simulink model "AGS_TFM_modelo_Aire_PI_descentralizado_clasico"  (R2025b)
settings: Solver=ode23tb  StartTime=0.0  StopTime=320  MaxStep=0.05  RelTol=1e-3
values from neighbouring files (symbols this model uses):
  k_Faraday_air = N_cells * M_O2 / (4 * F * Y_O2_air)    (= 0.000128302952219)    [AGS_base_subsitema_aire_SIMULINK.m]
  k_mref = lambda_air * k_Faraday_air    (= 0.000230945313994)    [AGS_base_subsitema_aire_SIMULINK.m]
  k_stack = 1.56e6    (= 1560000)    [AGS_base_subsitema_aire_SIMULINK.m]
  k_valve_max = 4e-4    (= 0.0004)    [AGS_base_subsitema_aire_SIMULINK.m]
  mdot_table_gs = [mdot_0_gs;mdot_40_tab; mdot_60_tab;          mdot_80_tab; mdot_100_tab; mdot_120_tab]    [AGS_init_mapa_compresor_2D.m]
  N_bp = [0 40000 60000 80000 100000 120000]    [AGS_init_mapa_compresor_2D.m]
  p_amb = 101325    [AGS_base_subsitema_aire_SIMULINK.m]
  PR_bp = 1.00:0.025:3.50    [AGS_init_mapa_compresor_2D.m]
  R_air = 287    [AGS_base_subsitema_aire_SIMULINK.m]
  T_air = 298.15    [AGS_base_subsitema_aire_SIMULINK.m]
  tau_N = 2.0 / 2.303    (= 0.868432479375)    [AGS_base_subsitema_aire_SIMULINK.m]
  V_eq = 0.01664    [AGS_base_subsitema_aire_SIMULINK.m]
libraries: slpidlib x2
settings Model: SimulationMode=accelerator  Creator=agonz  LastModifiedBy=agonz
settings DataIOCC: SaveOutput=off

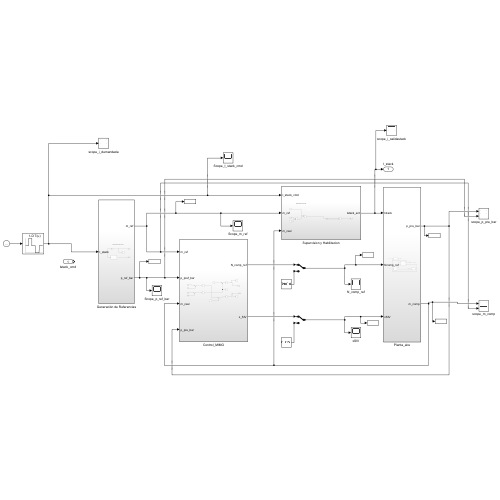
[thumbnail: Simulink's stored preview of the top-level diagram]
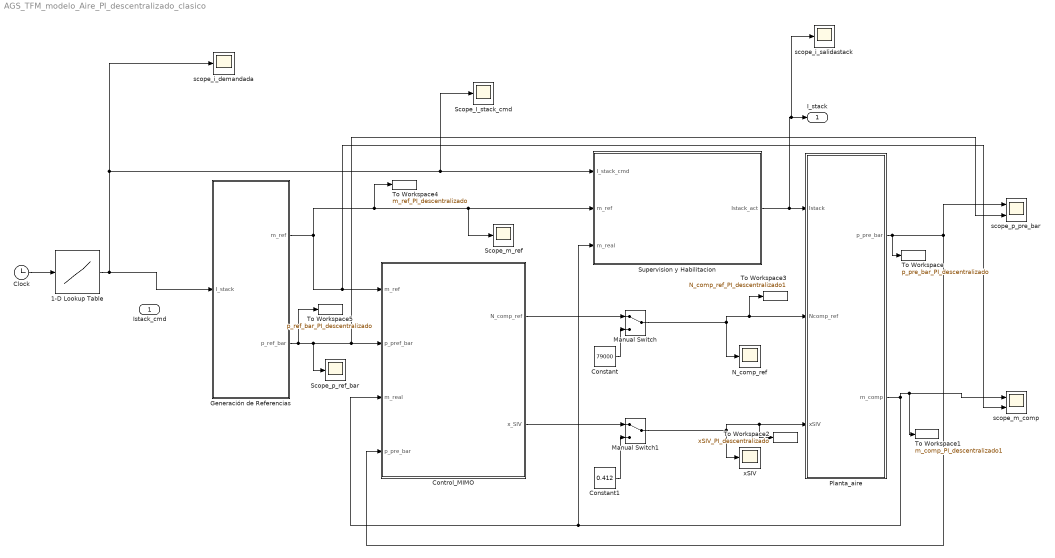
== system AGS_TFM_modelo_Aire_PI_descentralizado_clasico ==
  Istack_cmd : Inport
  1-D Lookup Table : Lookup_n-D  NumberOfTableDimensions=1  BreakpointsForDimension1=[0 40 43 90 93 140 143 200 203 250]  Table=[400 400 430 430 400 400 370 370 400 400]  InternalRulePriority=Speed  RndMeth=Simplest
  Clock : Clock
  Constant : Constant  Value=79000
  Constant1 : Constant  Value=0.412
  Control_MIMO : Subsystem
  Generación de Referencias : Subsystem
  Manual Switch : ManualSwitch
  Manual Switch1 : ManualSwitch
  N_comp_ref : Scope
      settings: ActiveDisplayYMinimum=64304.554984571354  ActiveDisplayYMaximum=126188.38277949208  DataLoggingVariableName=ScopeData6
  Planta_aire : Subsystem
  Scope_I_stack_cmd : Scope
      settings: ActiveDisplayYMinimum=-49.999999999999986  ActiveDisplayYMaximum=450  DataLoggingVariableName=ScopeData13
  Scope_m_ref : Scope
      settings: ActiveDisplayYMinimum=-0.011547265699688891  ActiveDisplayYMaximum=0.10392539129720003  DataLoggingVariableName=ScopeData9
  Scope_p_ref_bar : Scope
      settings: ActiveDisplayYMinimum=0.98812500000000014  ActiveDisplayYMaximum=1.856875  DataLoggingVariableName=ScopeData12
  Supervision y Habilitacion : Subsystem
  To Workspace : ToWorkspace  VariableName=p_pre_bar_PI_descentralizado  SaveFormat=Timeseries  SampleTime=-1
  To Workspace1 : ToWorkspace  VariableName=m_comp_PI_descentralizado1  SaveFormat=Timeseries  SampleTime=-1
  To Workspace2 : ToWorkspace  VariableName=xSIV_PI_descentralizado  SaveFormat=Timeseries  SampleTime=-1
  To Workspace3 : ToWorkspace  VariableName=N_comp_ref_PI_descentralizado1  SaveFormat=Timeseries  SampleTime=-1
  To Workspace4 : ToWorkspace  VariableName=m_ref_PI_descentralizado  SaveFormat=Timeseries  SampleTime=-1
  To Workspace5 : ToWorkspace  VariableName=p_ref_bar_PI_descentralizado  SaveFormat=Timeseries  SampleTime=-1
  scope_i_demandada : Scope
      settings: ActiveDisplayYMinimum=358.75  ActiveDisplayYMaximum=471.25  DataLoggingVariableName=ScopeData4
  scope_i_salidastack : Scope
      settings: ActiveDisplayYMinimum=-49.999999999999986  ActiveDisplayYMaximum=450  DataLoggingVariableName=ScopeData5
  scope_m_comp : Scope  NumInputPorts=2
      settings: TimeSpan=320  ActiveDisplayYMinimum=0.079577939696406835  ActiveDisplayYMaximum=0.10275653440906531
  scope_p_pre_bar : Scope  NumInputPorts=2
      settings: ActiveDisplayYMinimum=0.82562264109890293  ActiveDisplayYMaximum=2.6978636218977288
  xSIV : Scope
      settings: ActiveDisplayYMinimum=0.35571607291679863  ActiveDisplayYMaximum=0.82557864138077064  DataLoggingVariableName=ScopeData14
  I_stack : Outport
  wires:
  Planta_aire/1(p_pre_bar) -> To Workspace/1, scope_p_pre_bar/1, Control_MIMO/4(p_pre_bar)
  Supervision y Habilitacion/1(Istack_act) -> scope_i_salidastack/1, I_stack/1, Planta_aire/1(Istack)
  Generación de Referencias/1(m_ref) -> scope_m_comp/2, Control_MIMO/1(m_ref), To Workspace4/1, Scope_m_ref/1, Supervision y Habilitacion/2(m_ref)
  Generación de Referencias/2(p_ref_bar) -> To Workspace5/1, Scope_p_ref_bar/1, scope_p_pre_bar/2, Control_MIMO/2(p_pref_bar)
  Planta_aire/2(m_comp) -> To Workspace1/1, scope_m_comp/1, Control_MIMO/3(m_real), Supervision y Habilitacion/3(m_real)
  1-D Lookup Table/1 -> Scope_I_stack_cmd/1, Supervision y Habilitacion/1(I_stack_cmd), scope_i_demandada/1, Generación de Referencias/1(I_stack)
  Clock/1 -> 1-D Lookup Table/1
  Control_MIMO/1(N_comp_ref) -> Manual Switch/1
  Manual Switch/1 -> To Workspace3/1, Planta_aire/2(Ncomp_ref), N_comp_ref/1
  Control_MIMO/2(x_SIV) -> Manual Switch1/1
  Manual Switch1/1 -> xSIV/1, To Workspace2/1, Planta_aire/3(xSIV)
  Constant/1 -> Manual Switch/2
  Constant1/1 -> Manual Switch1/2

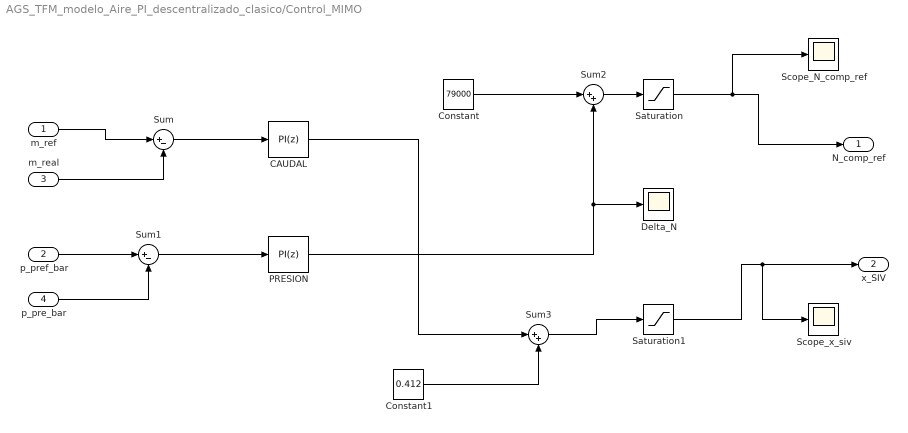
== system AGS_TFM_modelo_Aire_PI_descentralizado_clasico/Control_MIMO ==
  m_ref : Inport
  p_pref_bar : Inport  Port=2
  m_real : Inport  Port=3
  p_pre_bar : Inport  Port=4
  CAUDAL : slpidlib/PID Controller  Controller=PI  Form=Parallel  TimeDomain=Discrete-time  UseExternalTs=off  SampleTime=0.05  IntegratorMethod=Forward Euler  FilterMethod=Forward Euler  ControllerParametersSource=internal  P=0.131163  I=5.246523  UseKiTs=off  D=0  UseExternalDerivativeSource=off  N=100  UseFilter=on  TunerSelectOption=Transfer Function Based (PID Tuner App)  InitialConditionSource=internal  InitialConditionForIntegrator=0  InitialConditionForFilter=0  DifferentiatorICPrevScaledInput=0  ExternalReset=none  TrackingMode=off  Kt=1  LimitOutput=off  SatLimitsSource=internal  UpperSaturationLimit=inf  LowerSaturationLimit=-inf  LinearizeAsGain=off  AntiWindupMode=none  Kb=1  LimitIntegrator=off  UpperIntegratorSaturationLimit=inf  LowerIntegratorSaturationLimit=-inf  POutMin=[]  POutMax=[]  IOutMin=[]  IOutMax=[]  DOutMin=[]  DOutMax=[]  NOutMin=[]  NOutMax=[]  SumOutMin=[]  SumOutMax=[]  SaturationOutMin=[]  SaturationOutMax=[]  PParamMin=[]  PParamMax=[]  IParamMin=[]  IParamMax=[]  DParamMin=[]  DParamMax=[]  NParamMin=[]  NParamMax=[]  KbParamMin=[]  KbParamMax=[]  KtParamMin=[]  KtParamMax=[]  KbOutMin=[]  KbOutMax=[]  KtOutMin=[]  KtOutMax=[]  IntegratorOutMin=[]  IntegratorOutMax=[]  FilterOutMin=[]  FilterOutMax=[]  SumI1OutMin=[]  SumI1OutMax=[]  SumI2OutMin=[]  SumI2OutMax=[]  SumI3OutMin=[]  SumI3OutMax=[]  SumI4OutMin=[]  SumI4OutMax=[]  SumDOutMin=[]  SumDOutMax=[]  DifferentiatorOutMin=[]  DifferentiatorOutMax=[]  FilterDiffOutCoefMin=[]  FilterDiffOutCoefMax=[]  ReciprocalOutMin=[]  ReciprocalOutMax=[]  SumDenOutMin=[]  SumDenOutMax=[]  SumNumOutMin=[]  SumNumOutMax=[]  DivideOutMin=[]  DivideOutMax=[]  UdiffTsProdOutMin=[]  UdiffTsProdOutMax=[]  NTsProdOutMin=[]  NTsProdOutMax=[]  UintegralTsProdOutMin=[]  UintegralTsProdOutMax=[]  UngainTsProdOutMin=[]  UngainTsProdOutMax=[]  ClampingZeroOutDataTypeStr=Inherit: Inherit via back propagation  ClampingZeroOutMin=[]  ClampingZeroOutMax=[]  FilterDenConstantOutDataTypeStr=Inherit: Inherit via back propagation  FilterDenConstantOutMin=[]  FilterDenConstantOutMax=[]  PCopyOutDataTypeStr=Inherit: Inherit via back propagation  PCopyOutMin=[]  PCopyOutMax=[]  NCopyOutDataTypeStr=Inherit: Inherit via back propagation  NCopyOutMin=[]  NCopyOutMax=[]  IntegratorContinuousStateAttributes=''  IntegratorStateMustResolveToSignalObject=off  IntegratorRTWStateStorageClass=Auto  FilterContinuousStateAttributes=''  FilterStateMustResolveToSignalObject=off  FilterRTWStateStorageClass=Auto  ParallelPVariant=InternalParameters  IdealPVariant=Disabled  IVariant=InternalParameters  DVariant=Disabled  IntegratorVariant=Discrete  SatVariant=Disabled  AWVariant=Passthrough  PCopyVariant=Disabled  TRVariant=Disabled  FdbkBlocksVariant=Forward  IdealPFdbkVariant=Disabled  SatFdbkVariant=Disabled  DerivativeFilterVariant=Disabled  NVariant=Disabled  NCopyVariant=Disabled_SignalSpec  FilterICVariant=Disabled  IntegratorICVariant=InternalICs  ExternalResetVariant=Disabled  TRSumVariant=Passthrough  SumFdbkVariant=Disabled  SumVariant=Sum_PI  TsampFilterVariant=InternalTs  TsampNgainVariant=Passthrough  TsampIntegralVariant=Disabled_SignalSpec  ExternalSaturationOutDataTypeStr=Inherit: Same as second input  DerivativeSourceVariant=Disabled  PreIntVariant=InternalPreInt
      settings: LibrarySourceBlock=simulink/Discrete/Discrete PID Controller
  Constant : Constant  Value=79000
  Constant1 : Constant  Value=0.412
  Delta_N : Scope
      settings: ActiveDisplayYMinimum=-18781.831099261035  ActiveDisplayYMaximum=83965.8575339835  DataLoggingVariableName=ScopeData7
  PRESION : slpidlib/PID Controller  Controller=PI  Form=Parallel  TimeDomain=Discrete-time  UseExternalTs=off  SampleTime=0.05  IntegratorMethod=Forward Euler  FilterMethod=Forward Euler  ControllerParametersSource=internal  P=73897.888850  I=150636.822218  UseKiTs=off  D=0  UseExternalDerivativeSource=off  N=100  UseFilter=on  TunerSelectOption=Transfer Function Based (PID Tuner App)  InitialConditionSource=internal  InitialConditionForIntegrator=0  InitialConditionForFilter=0  DifferentiatorICPrevScaledInput=0  ExternalReset=none  TrackingMode=off  Kt=1  LimitOutput=off  SatLimitsSource=internal  UpperSaturationLimit=inf  LowerSaturationLimit=-inf  LinearizeAsGain=off  AntiWindupMode=none  Kb=1  LimitIntegrator=off  UpperIntegratorSaturationLimit=inf  LowerIntegratorSaturationLimit=-inf  POutMin=[]  POutMax=[]  IOutMin=[]  IOutMax=[]  DOutMin=[]  DOutMax=[]  NOutMin=[]  NOutMax=[]  SumOutMin=[]  SumOutMax=[]  SaturationOutMin=[]  SaturationOutMax=[]  PParamMin=[]  PParamMax=[]  IParamMin=[]  IParamMax=[]  DParamMin=[]  DParamMax=[]  NParamMin=[]  NParamMax=[]  KbParamMin=[]  KbParamMax=[]  KtParamMin=[]  KtParamMax=[]  KbOutMin=[]  KbOutMax=[]  KtOutMin=[]  KtOutMax=[]  IntegratorOutMin=[]  IntegratorOutMax=[]  FilterOutMin=[]  FilterOutMax=[]  SumI1OutMin=[]  SumI1OutMax=[]  SumI2OutMin=[]  SumI2OutMax=[]  SumI3OutMin=[]  SumI3OutMax=[]  SumI4OutMin=[]  SumI4OutMax=[]  SumDOutMin=[]  SumDOutMax=[]  DifferentiatorOutMin=[]  DifferentiatorOutMax=[]  FilterDiffOutCoefMin=[]  FilterDiffOutCoefMax=[]  ReciprocalOutMin=[]  ReciprocalOutMax=[]  SumDenOutMin=[]  SumDenOutMax=[]  SumNumOutMin=[]  SumNumOutMax=[]  DivideOutMin=[]  DivideOutMax=[]  UdiffTsProdOutMin=[]  UdiffTsProdOutMax=[]  NTsProdOutMin=[]  NTsProdOutMax=[]  UintegralTsProdOutMin=[]  UintegralTsProdOutMax=[]  UngainTsProdOutMin=[]  UngainTsProdOutMax=[]  ClampingZeroOutDataTypeStr=Inherit: Inherit via back propagation  ClampingZeroOutMin=[]  ClampingZeroOutMax=[]  FilterDenConstantOutDataTypeStr=Inherit: Inherit via back propagation  FilterDenConstantOutMin=[]  FilterDenConstantOutMax=[]  PCopyOutDataTypeStr=Inherit: Inherit via back propagation  PCopyOutMin=[]  PCopyOutMax=[]  NCopyOutDataTypeStr=Inherit: Inherit via back propagation  NCopyOutMin=[]  NCopyOutMax=[]  IntegratorContinuousStateAttributes=''  IntegratorStateMustResolveToSignalObject=off  IntegratorRTWStateStorageClass=Auto  FilterContinuousStateAttributes=''  FilterStateMustResolveToSignalObject=off  FilterRTWStateStorageClass=Auto  ParallelPVariant=InternalParameters  IdealPVariant=Disabled  IVariant=InternalParameters  DVariant=Disabled  IntegratorVariant=Discrete  SatVariant=Disabled  AWVariant=Passthrough  PCopyVariant=Disabled  TRVariant=Disabled  FdbkBlocksVariant=Forward  IdealPFdbkVariant=Disabled  SatFdbkVariant=Disabled  DerivativeFilterVariant=Disabled  NVariant=Disabled  NCopyVariant=Disabled_SignalSpec  FilterICVariant=Disabled  IntegratorICVariant=InternalICs  ExternalResetVariant=Disabled  TRSumVariant=Passthrough  SumFdbkVariant=Disabled  SumVariant=Sum_PI  TsampFilterVariant=InternalTs  TsampNgainVariant=Passthrough  TsampIntegralVariant=Disabled_SignalSpec  ExternalSaturationOutDataTypeStr=Inherit: Same as second input  DerivativeSourceVariant=Disabled  PreIntVariant=InternalPreInt
      settings: LibrarySourceBlock=simulink/Discrete/Discrete PID Controller
  Saturation : Saturate  UpperLimit=120000  LowerLimit=0
  Saturation1 : Saturate  UpperLimit=1  LowerLimit=0
  Scope_N_comp_ref : Scope
      settings: ActiveDisplayYMinimum=64304.554984571354  ActiveDisplayYMaximum=126188.38277949208  DataLoggingVariableName=ScopeData2
  Scope_x_siv : Scope
      settings: ActiveDisplayYMinimum=0.37668091218124344  ActiveDisplayYMaximum=0.62413168911243422  DataLoggingVariableName=ScopeData3
  Sum : Sum  Inputs=|+-
  Sum1 : Sum  Inputs=|+-
  Sum2 : Sum  Inputs=|++
  Sum3 : Sum  Inputs=|++
  N_comp_ref : Outport
  x_SIV : Outport  Port=2
  wires:
  m_real/1 -> Sum/2
  m_ref/1 -> Sum/1
  p_pref_bar/1 -> Sum1/1
  p_pre_bar/1 -> Sum1/2
  Sum/1 -> CAUDAL/1
  Sum1/1 -> PRESION/1
  Constant/1 -> Sum2/1
  Sum2/1 -> Saturation/1
  PRESION/1 -> Delta_N/1, Sum2/2
  Constant1/1 -> Sum3/2
  CAUDAL/1 -> Sum3/1
  Sum3/1 -> Saturation1/1
  Saturation/1 -> Scope_N_comp_ref/1, N_comp_ref/1
  Saturation1/1 -> Scope_x_siv/1, x_SIV/1

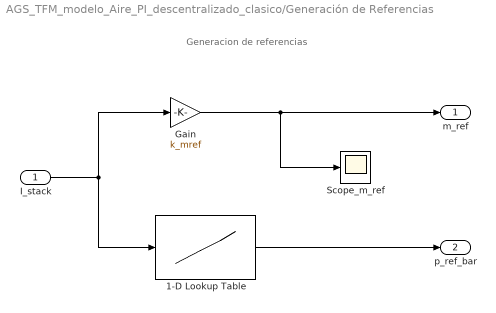
== system AGS_TFM_modelo_Aire_PI_descentralizado_clasico/Generación de Referencias ==
  note: Generacion de referencias
  I_stack : Inport
  1-D Lookup Table : Lookup_n-D  NumberOfTableDimensions=1  BreakpointsForDimension1=[30;50;75;100;125;150;200;250;300;350;400;450;500;525;550;570]  Table=[1.09;1.10;1.11;1.12;1.15;1.18;1.25;1.35;1.46;1.61;1.77;1.96;2.17;2.28;2.40;2.50]  InternalRulePriority=Speed  RndMeth=Simplest
  Gain : Gain  Gain=k_mref
  Scope_m_ref : Scope
      settings: ActiveDisplayYMinimum=-1  ActiveDisplayYMaximum=1  DataLoggingVariableName=ScopeData8
  m_ref : Outport
  p_ref_bar : Outport  Port=2
  wires:
  1-D Lookup Table/1 -> p_ref_bar/1
  I_stack/1 -> 1-D Lookup Table/1, Gain/1
  Gain/1 -> Scope_m_ref/1, m_ref/1

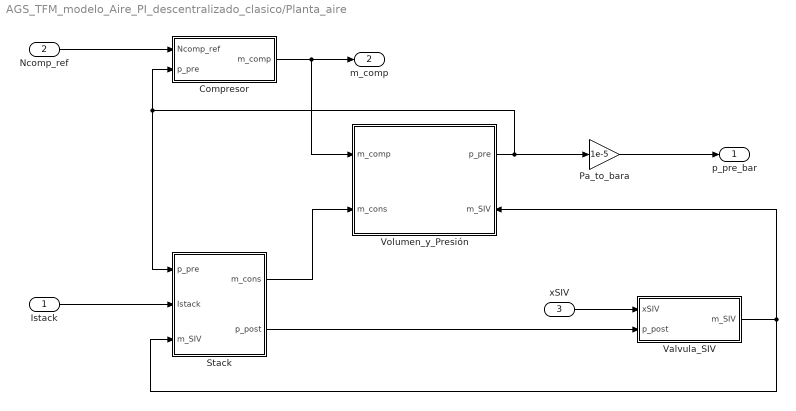
== system AGS_TFM_modelo_Aire_PI_descentralizado_clasico/Planta_aire ==
  Istack : Inport
  Ncomp_ref : Inport  Port=2
  xSIV : Inport  Port=3
  Compresor : Subsystem
  Pa_to_bara : Gain  Gain=1e-5
  Stack : Subsystem
  Valvula_SIV : Subsystem
  Volumen_y_Presión : Subsystem
      settings: PortSchema="{\"entries\":[{\"content\":{\"sides\":[{\"content\":{\"connectorIds\":[\"In1\",\"In2\"]},\"type\":\"ConnectorPlacement.EquallySpacedRectSide\",\"uuid\":\"9adf6fab-0cc5-4123-839b-d242686084c8\"},{\"content\":{\"connectorIds\":[\"Out1\",\"In3\"],\"side\":\"RIGHT\"},\"type\":\"ConnectorPlacement.EquallySpacedRectSide\",\"uuid\":\"fb019ae7-8558-4add-b28a-d89906b0a695\"},{\"content\":{\"side\":\"TOP\"},\"type\":\"ConnectorPlacement.EquallySpacedRectSide\",\"uuid\":\"307403d9-68c4-48bc-9646-6dcb13d017bf\"}]},\"type\":\"ConnectorPlacement.EquallySpacedConnector\",\"uuid\":\"1e49d5e7-eb04-450d-88b2-45a0c8b49afe\"}],\"packageUris\":[\"http://schema.mathworks.com/mf0/Connector/R2020b\"],\"version\":\"1.0\"}"
  p_pre_bar : Outport
  m_comp : Outport  Port=2
  wires:
  Stack/1(m_cons) -> Volumen_y_Presión/2(m_cons)
  Volumen_y_Presión/1(p_pre) -> Pa_to_bara/1, Compresor/2(p_pre), Stack/1(p_pre)
  Valvula_SIV/1(m_SIV) -> Volumen_y_Presión/3(m_SIV), Stack/3(m_SIV)
  Ncomp_ref/1 -> Compresor/1(Ncomp_ref)
  Compresor/1(m_comp) -> m_comp/1, Volumen_y_Presión/1(m_comp)
  Istack/1 -> Stack/2(Istack)
  xSIV/1 -> Valvula_SIV/1(xSIV)
  Stack/2(p_post) -> Valvula_SIV/2(p_post)
  Pa_to_bara/1 -> p_pre_bar/1

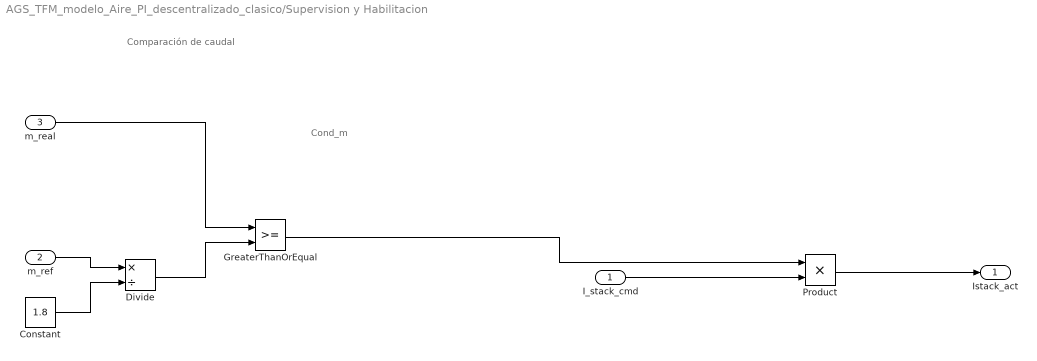
== system AGS_TFM_modelo_Aire_PI_descentralizado_clasico/Supervision y Habilitacion ==
  note: Cond_m
  note: Comparación de caudal
  I_stack_cmd : Inport
  m_ref : Inport  Port=2
  m_real : Inport  Port=3
  Constant : Constant  Value=1.8
  Divide : Product  Inputs=*/
  GreaterThanOrEqual : RelationalOperator  OutDataTypeStr=boolean  RndMeth=Simplest  InputSameDT=off
  Product : Product
  Istack_act : Outport
  wires:
  GreaterThanOrEqual/1 -> Product/1
  I_stack_cmd/1 -> Product/2
  Product/1 -> Istack_act/1
  m_real/1 -> GreaterThanOrEqual/1
  m_ref/1 -> Divide/1
  Constant/1 -> Divide/2
  Divide/1 -> GreaterThanOrEqual/2

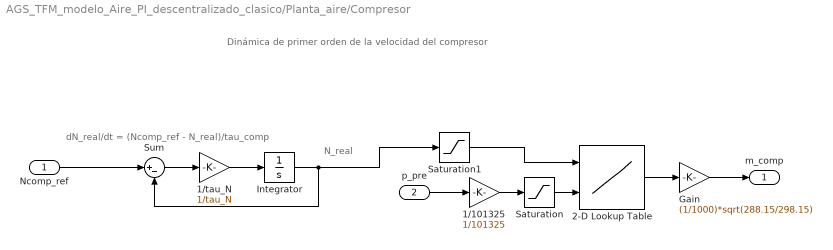
== system AGS_TFM_modelo_Aire_PI_descentralizado_clasico/Planta_aire/Compresor ==
  note: dN_real/dt = (Ncomp_ref - N_real)/tau_comp
  note: Dinámica de primer orden de la velocidad del compresor
  note: N_real
  Ncomp_ref : Inport
  p_pre : Inport  Port=2
  1/101325 : Gain  Gain=1/101325
  1/tau_N : Gain  Gain=1/tau_N
  2-D Lookup Table : Lookup_n-D  BreakpointsForDimension1=N_bp  BreakpointsForDimension2=PR_bp  Table=mdot_table_gs  InternalRulePriority=Speed  RndMeth=Simplest
      settings: InputPortMap=u0,u1
  Gain : Gain  Gain=(1/1000)*sqrt(288.15/298.15)
  Integrator : Integrator
  Saturation : Saturate  UpperLimit=3.5  LowerLimit=1.5
  Saturation1 : Saturate  UpperLimit=120000  LowerLimit=0
  Sum : Sum  Inputs=|+-
  m_comp : Outport
  wires:
  Ncomp_ref/1 -> Sum/1
  Sum/1 -> 1/tau_N/1
  1/tau_N/1 -> Integrator/1
  Integrator/1 -> Saturation1/1, Sum/2
  p_pre/1 -> 1/101325/1
  1/101325/1 -> Saturation/1
  Saturation/1 -> 2-D Lookup Table/2
  Saturation1/1 -> 2-D Lookup Table/1
  2-D Lookup Table/1 -> Gain/1
  Gain/1 -> m_comp/1

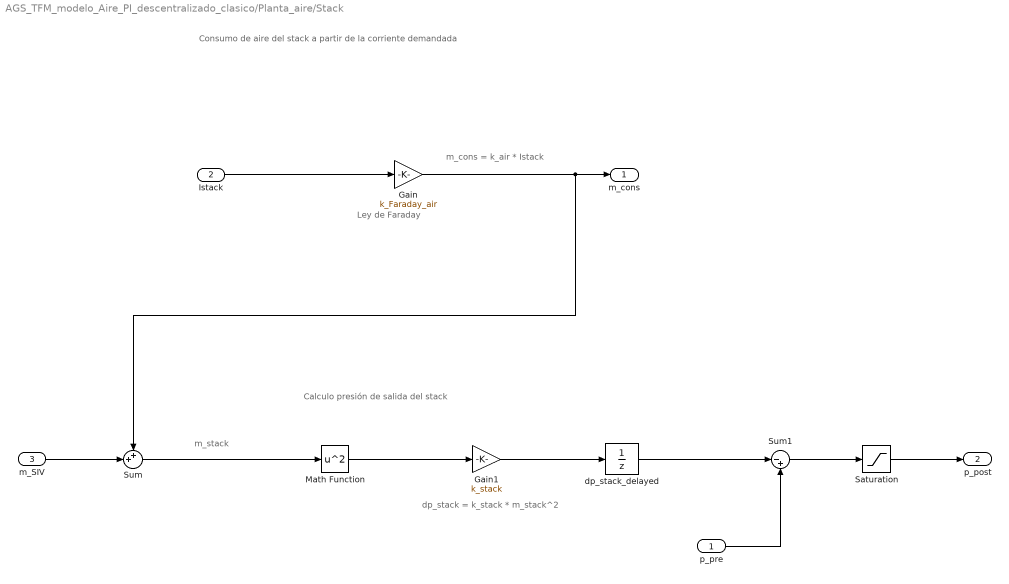
== system AGS_TFM_modelo_Aire_PI_descentralizado_clasico/Planta_aire/Stack ==
  note: m_stack
  note: dp_stack = k_stack * m_stack^2
  note: Calculo presión de salida del stack
  note: m_cons = k_air * Istack
  note: Ley de Faraday
  note: Consumo de aire del stack a partir de la corriente demandada
  p_pre : Inport
  Istack : Inport  Port=2
  m_SIV : Inport  Port=3
  Gain : Gain  Gain=k_Faraday_air
  Gain1 : Gain  Gain=k_stack
  Math Function : Math  Operator=square
  Saturation : Saturate  UpperLimit=1e12  LowerLimit=p_amb  ZeroCross=off
  Sum : Sum  Inputs=++|
  Sum1 : Sum  Inputs=|-+
  dp_stack_delayed : UnitDelay  SampleTime=-1  HasFrameUpgradeWarning=on
  m_cons : Outport
  p_post : Outport  Port=2
  wires:
  Istack/1 -> Gain/1
  Gain/1 -> Sum/1, m_cons/1
  Math Function/1 -> Gain1/1
  Gain1/1 -> dp_stack_delayed/1
  m_SIV/1 -> Sum/2
  Sum/1 -> Math Function/1
  dp_stack_delayed/1 -> Sum1/1
  p_pre/1 -> Sum1/2
  Sum1/1 -> Saturation/1
  Saturation/1 -> p_post/1

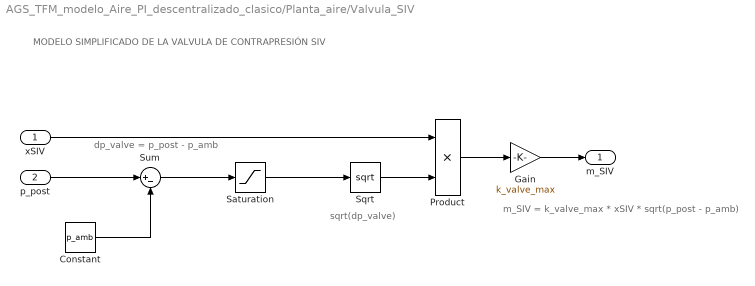
== system AGS_TFM_modelo_Aire_PI_descentralizado_clasico/Planta_aire/Valvula_SIV ==
  note: m_SIV = k_valve_max * xSIV * sqrt(p_post - p_amb)
  note: sqrt(dp_valve)
  note: dp_valve = p_post - p_amb
  note: MODELO SIMPLIFICADO DE LA VALVULA DE CONTRAPRESIÓN SIV
  xSIV : Inport
  p_post : Inport  Port=2
  Constant : Constant  Value=p_amb
  Gain : Gain  Gain=k_valve_max
  Product : Product
  Saturation : Saturate  UpperLimit=1e12  LowerLimit=0  ZeroCross=off
  Sqrt : Sqrt
  Sum : Sum  Inputs=|+-
  m_SIV : Outport
  wires:
  p_post/1 -> Sum/1
  Constant/1 -> Sum/2
  xSIV/1 -> Product/1
  Product/1 -> Gain/1
  Gain/1 -> m_SIV/1
  Sqrt/1 -> Product/2
  Sum/1 -> Saturation/1
  Saturation/1 -> Sqrt/1

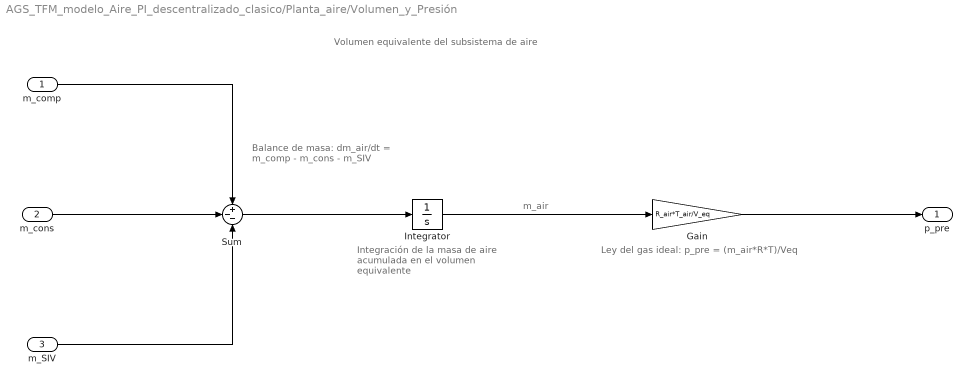
== system AGS_TFM_modelo_Aire_PI_descentralizado_clasico/Planta_aire/Volumen_y_Presión ==
  note: m_air
  note: Volumen equivalente del subsistema de aire
  note: Ley del gas ideal: p_pre = (m_air*R*T)/Veq
  note: Integración de la masa de aire acumulada en el volumen equivalente
  note: Balance de masa: dm_air/dt = m_comp - m_cons - m_SIV
  m_comp : Inport
  m_cons : Inport  Port=2
  m_SIV : Inport  Port=3
  Gain : Gain  Gain=R_air*T_air/V_eq
  Integrator : Integrator  InitialCondition=0.02
  Sum : Sum  Inputs=+--
  p_pre : Outport
  wires:
  m_comp/1 -> Sum/1
  m_cons/1 -> Sum/2
  m_SIV/1 -> Sum/3
  Integrator/1 -> Gain/1
  Gain/1 -> p_pre/1
  Sum/1 -> Integrator/1
